simulink model "MultirotorSimPx4v1_8FPHT"  (R2020b)
settings: Solver=VariableStepAuto  StartTime=0.0  StopTime=Simulation.T_END  MaxStep=Simulation.TS_MAX  RelTol=1e-3  EnableMultiTasking=on
PreLoadFcn:
  | % InitializeParameters;
undefined symbols (not defined in the file): Aero, Ctrl, Initial, Motor, Uav, Wind
libraries: QuaternionLibrary x11, simulink_extras x2
(part 2 of 2)

== matlab function MultirotorSimPx4v1_8FPHT/Quadrotor Euler Model/compute VBody ==
  data: eta input; VBody output; xiDot input
function VBody = computeVBody(eta, xiDot)
%#codegen

sphi = sin(eta(1));
sTheta = sin(eta(2));
sPsi = sin(eta(3));
cPhi = cos(eta(1));
cTheta = cos(eta(2));
cPsi = cos(eta(3));

R = [ cPsi*cTheta, cPsi*sTheta*sphi-sPsi*cPhi, cPsi*sTheta*cPhi+sPsi*sphi;
	  sPsi*cTheta, sPsi*sTheta*sphi+cPsi*cPhi, sPsi*sTheta*cPhi-cPsi*sphi;
     -sTheta,      cTheta*sphi,                cTheta*cPhi+sPsi*sphi];

VBody = R'*xiDot;

== matlab function MultirotorSimPx4v1_8FPHT/L2 norm ==
  data: u input; y output
function y = l2norm( u )
    y = sqrt( dot(u, u) );
end

== matlab function MultirotorSimPx4v1_8FPHT/Motor model 2/Compute Sph ==
  data: V_appBody input; polar output
function polar  = computeSph(V_appBody)
%#codegen

% Convert from polar to spherical coordinates
[ azimuth, elevation, radius ] = cart2sph( V_appBody(1), V_appBody(2), V_appBody(3) );

polar = [azimuth; elevation; radius];

== matlab function MultirotorSimPx4v1_8FPHT/Motor model 2/Individual motor force//torque ==
  data: omega input; TMotorIndividual output; omegaDot input; polarC input; Motor parameter; Uav parameter; tauMotorIndividual output; Aero parameter
function [TMotorIndividual, tauMotorIndividual] = motorIndividual( ...
    omega, omegaDot, polarC, Motor, Uav, Aero)
%#codegen
    alpha = polarC(2);
    beta  = polarC(1);
    U     = polarC(3);

    % Make assertions to avoid code generation errors
    %assert(Uav.N_ROTORS < 16);
    % Uav.N_ROTORS = 4;

    % Output
    % TMotorIndividual   = zeros(3, Uav.N_ROTORS);
    %tauMotorIndividual = zeros(3, Uav.N_ROTORS);

    %% Thrust and differential torque

    % Concatenated motor force/torque vectors in respective motor frame
    % eg. TMotor = [TMotor1, TMotor2, ..., TMotorN]
    % where: - N is the number of rotors
    %        - TMotorx (x ∈ [1,2,...,N]) is the thrust generated by motor x in
    %          its own frame of reference
    % For basic thrust model:
    % TMotorIndividual = [ zeros(2, Uav.N_ROTORS);
    %                      K * (omega'.^2) ];

    Cz2 = dot( Aero.Cz2.coefs, [alpha, 1]);
    p = Aero.Cz3.coefs;
    lambda = omega .* Uav.D_PROP / ( 2 * U );
    Cz3 = p(1) * sin(alpha) + p(2) * ( 1 - exp(-p(3).*lambda) ) .* sin(3*alpha) + ...
        p(4);
    p = Aero.Cx2.coefs;
    Cx2 = p(1) * ( 1 - exp(-p(2).*lambda) ) .* cos(alpha) + ...
          p(3) * ( 1 - exp(-p(4).*lambda) ) .* cos(3*alpha);
    Tz = -0.5 .* Uav.RHO_AIR .* omega'.^2 .* (Cz2) .* Uav.D_PROP^2 .* Uav.A_PROP - ... % Rotor thrust
          0.5 .* Uav.RHO_AIR .* (Cz3)' .* U .*  omega' .* Uav.D_PROP .* Uav.A_PROP;    % Rotor thrust correction
    Tx = -0.5 .* Uav.RHO_AIR .* (Cx2)' .* U .* omega' .* Uav.D_PROP .* Uav.A_PROP;
    TMotorIndividual = [ Tx.*cos(beta); Tx.*sin(beta); Tz ];

    tauMotorIndividual = [ 0*omega'; 0*omega'; % Avoid using zeros(1,Uav.N_ROTORS), which causes issues
        -Uav.ROTOR_DIRECTION .* ( Motor.B .* omega'.^2 + Motor.I_R_ZZ .* omegaDot' ) ];
end

== matlab function MultirotorSimPx4v1_8FPHT/Motor model 2/Combined motor force//torque ==
  data: TMotorIndividual input; TBody output size=3; tauMotorIndividual input; tauBody output size=3; omega input; nuBody input; Motor parameter; Uav parameter
function [TBody, tauBody] = motorCombined( TMotorIndividual,tauMotorIndividual,  ...
    omega, nuBody, Motor, Uav)
%#codegen
assert(Uav.N_ROTORS < 16);

% Initialise matrices to store motor force/torque vectors in body frame
TBodyIndividual   = zeros(3, Uav.N_ROTORS);
tauBodyIndividual = zeros(3, Uav.N_ROTORS);

% Calculate forces and moments from each motor in the body frame
for i = 1:Uav.N_ROTORS
    l = Uav.L(i);
    beta = Uav.BETA(i);
    
    % Matrix to compute torque applied by rotor thrust
 	L = [ 0,            0,            l*sin(beta);
          0,            0,           -l*cos(beta);
         -l*sin(beta),  l*cos(beta),  0 ];

	% Motor force/torque vectors in body frame
	TBodyIndividual(:,i) = Uav.R_MOTOR_TO_BODY(:,:,i) * ...
        TMotorIndividual(:,i);
	tauBodyIndividual(:,i) = Uav.R_MOTOR_TO_BODY(:,:,i) * ...
        tauMotorIndividual(:,i) + L * TBodyIndividual(:,i);
end

%% Gyroscopic moments

% Concatenated gyroscopic moments for each rotor
M_GBodyIndividual = zeros(3, Uav.N_ROTORS);
H_MMotorSeparate = zeros(3, Uav.N_ROTORS);

% Concatenated motor speeds in their respective frames
omegaMotor = [ zeros(2, Uav.N_ROTORS);
               Uav.ROTOR_DIRECTION .* omega' ];

for i = 1:Uav.N_ROTORS
    % Angular momentum in motor frame
    H_MMotorSeparate(:,i) = Motor.I_R(:,:,i) * omegaMotor(:,i);
    % Gyroscopic moment vectors in body frame
    M_GBodyIndividual(:,i) = cross( nuBody, ...
        Uav.R_MOTOR_TO_BODY(:,:,i) * H_MMotorSeparate(:,i) );
end

M_GBody = sum(M_GBodyIndividual, 2);

%% Total torque and moment

% Total force/torque in body frame
TBody = sum(TBodyIndividual, 2);
tauBody = sum(tauBodyIndividual, 2) - M_GBody;

end

== matlab function MultirotorSimPx4v1_8FPHT/Motor model 2/Motor rotational dynamics ==
  data: pwm input; omegaDot output; omega input; realPwm output
function [omegaDot, realPwm]  = motorRotDynamics( pwm, omega )
%#codegen

realPwm = (1000 * pwm + 1000);

rotorTimeConst = 7.006512e-02;
omegaRef = 0.84 * ( 7.969173e-1.*realPwm - 6.528579e2 );

omegaDot = (omegaRef - omega) / rotorTimeConst;
end

== matlab function MultirotorSimPx4v1_8FPHT/Quadrotor Euler Model/Equations of motion ==
  data: VBody input; VBodyDot output; nuBody input; eta input; etaDot input; TBody input size=3; tauBody input size=3; F_D input size=3; M_D input size=3; nuBodyDot output; Uav parameter; xiDDot output; etaDDot output
function [VBodyDot, nuBodyDot, xiDDot, etaDDot] = QuadrotorQuaternionModel(...
    VBody, nuBody, eta, etaDot, TBody, tauBody, F_D, M_D, Uav )
%#codegen

%% Rotation matrices
% Precompute sines and cosines
sPhi   = sin(eta(1));
sTheta = sin(eta(2));
sPsi   = sin(eta(3));
cPhi   = cos(eta(1));
cTheta = cos(eta(2));
cPsi   = cos(eta(3));
tTheta = tan(eta(2));

phiDot   = etaDot(1);
thetaDot = etaDot(2);

% Body frame to inertial frame
R = [cPsi*cTheta, cPsi*sTheta*sPhi-sPsi*cPhi, cPsi*sTheta*cPhi+sPsi*sPhi;
     sPsi*cTheta, sPsi*sTheta*sPhi+cPsi*cPhi, sPsi*sTheta*cPhi-cPsi*sPhi;
     -sTheta,     cTheta*sPhi,                cTheta*cPhi+sPsi*sPhi];

WInvertDot = [...
    0,  phiDot*cPhi*tTheta+thetaDot*sPhi/cTheta^2,    -phiDot*sPhi*cTheta+thetaDot*cPhi/cTheta^2;
    0, -phiDot*sPhi,                                  -phiDot*cPhi;
	0,  phiDot*cPhi/cTheta+phiDot*sPhi*tTheta/cTheta, -phiDot*sPhi/cTheta+thetaDot*cPhi*tTheta/cTheta];

WInvert = [1, sPhi*tTheta,  cPhi*tTheta;
           0, cPhi,        -sPhi;
           0, sPhi/cTheta,  cPhi/cTheta];


%% Moments and Forces
% Body frame accelerations
VBodyDot  = (1/Uav.M) * (R'*Uav.G + TBody - cross(nuBody, Uav.M*VBody) + F_D);
nuBodyDot = Uav.I \ (tauBody - cross(nuBody, Uav.I*nuBody) + M_D);

% Inertial frame accelerations
xiDDot = (1/Uav.M)*(Uav.G + R*TBody + R*F_D);
etaDDot = WInvertDot*nuBody + WInvert*nuBodyDot;

end

== matlab function MultirotorSimPx4v1_8FPHT/Pos Control1/MATLAB Function ==
  data: thr_sp input size=3; q_sp output; yaw_sp input; thrust_sp output
function [q_sp, thrust_sp] = thrustToAttitude( thr_sp, yaw_sp )

    yaw_body = yaw_sp;
    body_z = -thr_sp./norm(thr_sp);
    
    y_C = [ -sin(yaw_body); cos(yaw_body); 0 ];
    
    body_x = zeros(3,1);
    if body_z(3) > 0.000001
        body_x = cross( y_C, body_z );
        if ( body_z(3) < 0 )
            body_x = -body_x;
        end
        
        body_x = body_x ./ norm(body_x);
    else
        body_x(3) = 1;
    end
    
    body_y = cross( body_z, body_x );
    
    R_sp = [ body_x, body_y, body_z ];
    
    q_sp = from_dcm( R_sp );
    
    thrust_sp = -norm( thr_sp );
    
end

function data  = from_dcm( dcm )
% FROM_DCM Convert DCM to quaternion
% From https://github.com/PX4/Firmware/blob/master/src/lib/mathlib/math/Quaternion.hpp
    data = zeros(4,1);
    tr = dcm(1,1) + dcm(2,2) + dcm(3,3);
    if (tr > 0.0)
        s = sqrt(tr + 1.0);
        data(1) = s * 0.5;
        s = 0.5 / s;
        data(2) = (dcm(3,2) - dcm(2,3) ) * s;
        data(3) = (dcm(1,3) - dcm(3,1) ) * s;
        data(4) = (dcm(2,1) - dcm(1,2) ) * s;
    else
        % Find maximum diagonal element in dcm
        % store index in dcm_i
        dcm_i = 1;
        for i = 2:3 % (int i = 1; i < 3; i++)
            if ( dcm(i,i) > dcm(dcm_i,dcm_i) )
                dcm_i = i;
            end
        end
        dcm_j = rem( ( (dcm_i-1) + 1), 3) + 1;
        dcm_k = rem( ( (dcm_i-1) + 2), 3) + 1;
        s = sqrt( (dcm(dcm_i, dcm_i) - dcm(dcm_j, dcm_j) - ...
            dcm(dcm_k,dcm_k)) + 1.0 );
        data(dcm_i + 1) = s * 0.5;
        s = 0.5 / s;
        data(dcm_j + 1) = ( dcm(dcm_i,dcm_j) + dcm(dcm_j,dcm_i) ) * s;
        data(dcm_k + 1) = ( dcm(dcm_k,dcm_i) + dcm(dcm_i,dcm_k) ) * s;
        data(1) = ( dcm(dcm_k,dcm_j) - dcm(dcm_j,dcm_k) ) * s;
    end
end

== matlab function MultirotorSimPx4v1_8FPHT/Pos Control - base/MATLAB Function1 ==
  data: thr_sp input size=3; q_sp output; yaw_sp input; thrust_sp output
function [q_sp, thrust_sp] = thrustToAttitude( thr_sp, yaw_sp )

    yaw_body = yaw_sp;
    body_z = -thr_sp./norm(thr_sp);
    
    y_C = [ -sin(yaw_body); cos(yaw_body); 0 ];
    
    body_x = zeros(3,1);
    if body_z(3) > 0.000001
        body_x = cross( y_C, body_z );
        if ( body_z(3) < 0 )
            body_x = -body_x;
        end
        
        body_x = body_x ./ norm(body_x);
    else
        body_x(3) = 1;
    end
    
    body_y = cross( body_z, body_x );
    
    R_sp = [ body_x, body_y, body_z ];
    
    q_sp = from_dcm( R_sp );
    
    thrust_sp = -norm( thr_sp );
    
end

function data  = from_dcm( dcm )
% FROM_DCM Convert DCM to quaternion
% From https://github.com/PX4/Firmware/blob/master/src/lib/mathlib/math/Quaternion.hpp
    data = zeros(4,1);
    tr = dcm(1,1) + dcm(2,2) + dcm(3,3);
    if (tr > 0.0)
        s = sqrt(tr + 1.0);
        data(1) = s * 0.5;
        s = 0.5 / s;
        data(2) = (dcm(3,2) - dcm(2,3) ) * s;
        data(3) = (dcm(1,3) - dcm(3,1) ) * s;
        data(4) = (dcm(2,1) - dcm(1,2) ) * s;
    else
        % Find maximum diagonal element in dcm
        % store index in dcm_i
        dcm_i = 1;
        for i = 2:3 % (int i = 1; i < 3; i++)
            if ( dcm(i,i) > dcm(dcm_i,dcm_i) )
                dcm_i = i;
            end
        end
        dcm_j = rem( ( (dcm_i-1) + 1), 3) + 1;
        dcm_k = rem( ( (dcm_i-1) + 2), 3) + 1;
        s = sqrt( (dcm(dcm_i, dcm_i) - dcm(dcm_j, dcm_j) - ...
            dcm(dcm_k,dcm_k)) + 1.0 );
        data(dcm_i + 1) = s * 0.5;
        s = 0.5 / s;
        data(dcm_j + 1) = ( dcm(dcm_i,dcm_j) + dcm(dcm_j,dcm_i) ) * s;
        data(dcm_k + 1) = ( dcm(dcm_k,dcm_i) + dcm(dcm_i,dcm_k) ) * s;
        data(1) = ( dcm(dcm_k,dcm_j) - dcm(dcm_j,dcm_k) ) * s;
    end
end

== matlab function MultirotorSimPx4v1_8FPHT/Applied wind speed/Relative velocity ==
  data: nuBody input; Uav parameter; VMotorRelBody output
function VMotorRelBody = relativeMotorVelocity( nuBody , Uav )
%#codegen
    VMotorRelBody = cross( nuBody, Uav.L_VEC );
end

== matlab function MultirotorSimPx4v1_8FPHT/Applied wind speed/Compute V_app2 ==
  data: Q input; UBody output; U input size=3
function UBody = computeUBody(Q, U)
%#codegen

% Rotation matrix from Wind frame to Inertial frame
% Wind frame SEU, inertial frame NED
R_U = [1,  0, 0;
       0, -1, 0;
       0,  0, 1];
   
UBody = Q' * R_U * U;

== matlab function MultirotorSimPx4v1_8FPHT/Pos Control/MATLAB Function1 ==
  data: thr_sp input size=3; q_sp output; yaw_sp input; thrust_sp output
function [q_sp, thrust_sp] = thrustToAttitude( thr_sp, yaw_sp )

    yaw_body = yaw_sp;
    body_z = -thr_sp./norm(thr_sp);
    
    y_C = [ -sin(yaw_body); cos(yaw_body); 0 ];
    
    body_x = zeros(3,1);
    if body_z(3) > 0.000001
        body_x = cross( y_C, body_z );
        if ( body_z(3) < 0 )
            body_x = -body_x;
        end
        
        body_x = body_x ./ norm(body_x);
    else
        body_x(3) = 1;
    end
    
    body_y = cross( body_z, body_x );
    
    R_sp = [ body_x, body_y, body_z ];
    
    q_sp = from_dcm( R_sp );
    
    thrust_sp = -norm( thr_sp );
    
end

function data  = from_dcm( dcm )
% FROM_DCM Convert DCM to quaternion
% From https://github.com/PX4/Firmware/blob/master/src/lib/mathlib/math/Quaternion.hpp
    data = zeros(4,1);
    tr = dcm(1,1) + dcm(2,2) + dcm(3,3);
    if (tr > 0.0)
        s = sqrt(tr + 1.0);
        data(1) = s * 0.5;
        s = 0.5 / s;
        data(2) = (dcm(3,2) - dcm(2,3) ) * s;
        data(3) = (dcm(1,3) - dcm(3,1) ) * s;
        data(4) = (dcm(2,1) - dcm(1,2) ) * s;
    else
        % Find maximum diagonal element in dcm
        % store index in dcm_i
        dcm_i = 1;
        for i = 2:3 % (int i = 1; i < 3; i++)
            if ( dcm(i,i) > dcm(dcm_i,dcm_i) )
                dcm_i = i;
            end
        end
        dcm_j = rem( ( (dcm_i-1) + 1), 3) + 1;
        dcm_k = rem( ( (dcm_i-1) + 2), 3) + 1;
        s = sqrt( (dcm(dcm_i, dcm_i) - dcm(dcm_j, dcm_j) - ...
            dcm(dcm_k,dcm_k)) + 1.0 );
        data(dcm_i + 1) = s * 0.5;
        s = 0.5 / s;
        data(dcm_j + 1) = ( dcm(dcm_i,dcm_j) + dcm(dcm_j,dcm_i) ) * s;
        data(dcm_k + 1) = ( dcm(dcm_k,dcm_i) + dcm(dcm_i,dcm_k) ) * s;
        data(1) = ( dcm(dcm_k,dcm_j) - dcm(dcm_j,dcm_k) ) * s;
    end
end
